simulink model "ACC_COM"  (R2022b)
settings: configuration reference "ACC_AutosarConfig" (kept outside this file)
model workspace (MATLAB code in the model file):
  | cmdLim = Simulink.Parameter;
  | cmdLim.Value = 15;
  | cmdLim.Description = 'Limit for controlling the maximum surface command angle.';
  | cmdLim.Min = 0;
  | cmdLim.Max = 90;
  | cmdLim.DocUnits = 'deg';
  | 
  | dispGain = Simulink.Parameter;
  | dispGain.Value = 0.75;
  | dispGain.Description = 'Gain applied to the displacement error.';
  | dispGain.Min = 0;
  | dispGain.Max = [];
  | dispGain.DocUnits = 'deg/sec/deg';
  | 
  | dispLim = Simulink.Parameter;
  | dispLim.Value = 30;
  | dispLim.Description = 'Limit for controlling the maximum commanded angle.';
  | dispLim.Min = 0;
  | dispLim.Max = 180;
  | dispLim.DocUnits = 'deg';
  | 
  | intGain = Simulink.Parameter;
  | intGain.Value = 0.5;
  | intGain.Description = 'Gain applied to the integral error.';
  | intGain.Min = 0;
  | intGain.Max = [];
  | intGain.DocUnits = 'deg/sec/deg/sec';
  | 
  | intLim = Simulink.Parameter;
  | intLim.Value = 5;
  | intLim.Description = 'Limit for controlling the maximum commanded angle.';
  | intLim.Min = 0;
  | intLim.Max = 90;
  | intLim.DocUnits = 'deg';
  | 
  | rateGain = Simulink.Parameter;
  | rateGain.Value = 2;
  | rateGain.Description = 'Gain applied to the rate error.';
  | rateGain.Min = 0;
  | rateGain.Max = [];
  | rateGain.DocUnits = 'deg/deg/sec';
  | 
  | rateLim = Simulink.Parameter;
  | rateLim.Value = 6;
  | rateLim.Description = 'Limit for controlling the maximum commanded angle.';
  | rateLim.Min = 0;
  | rateLim.Max = 180;
  | rateLim.DocUnits = 'deg/sec';
  | 
  | hdgGain = Simulink.Parameter;
  | hdgGain.Value = 0.015;
values from neighbouring files (symbols this model uses):
  ACC_SampleTime = 0.01    [ACC_DD.sldd]
settings Model: RequirementInfo={} %GIDa_fe9045fd_0412_4b6e_8206_617cc20e6fde  DataDictionary=ACC_DD.sldd  FPTRunName=Active  Creator=MAAM  LastModifiedBy=MAAM
settings ConfigSetRef: SourceName=ACC_AutosarConfig

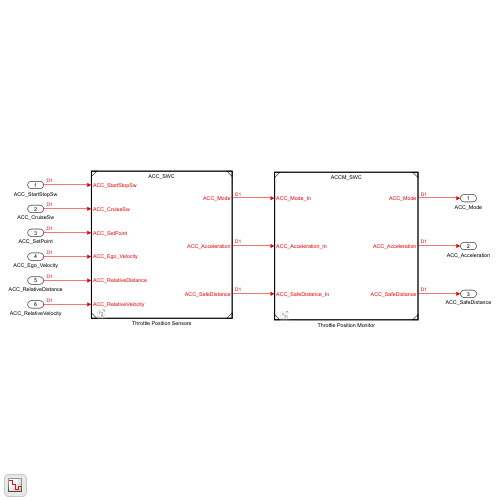
[thumbnail: Simulink's stored preview of the top-level diagram]
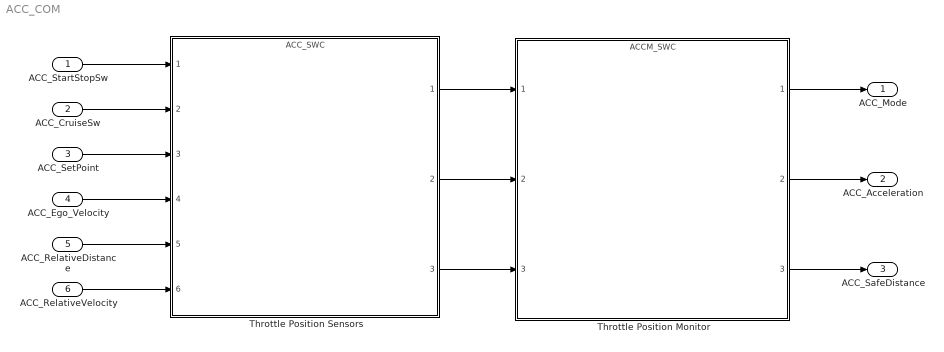
== system ACC_COM ==
  ACC_StartStopSw : Inport  OutDataTypeStr=boolean  SampleTime=ACC_SampleTime
  ACC_CruiseSw : Inport  Port=2  OutDataTypeStr=boolean  SampleTime=ACC_SampleTime
  ACC_SetPoint : Inport  Port=3  OutDataTypeStr=single  SampleTime=ACC_SampleTime
  ACC_Ego_Velocity : Inport  Port=4  OutDataTypeStr=single  SampleTime=ACC_SampleTime
  ACC_RelativeDistance : Inport  Port=5  OutDataTypeStr=single  SampleTime=ACC_SampleTime
  ACC_RelativeVelocity : Inport  Port=6  OutDataTypeStr=single  SampleTime=ACC_SampleTime
  Throttle Position Monitor : ModelReference  ModelNameDialog=ACCM_SWC.slx  SimulationMode=Normal  ModelReferenceVersion=1.7
  Throttle Position Sensors : ModelReference  ModelNameDialog=ACC_SWC.slx  SimulationMode=Normal  ModelReferenceVersion=1.6
  ACC_Mode : Outport
  ACC_Acceleration : Outport  Port=2
  ACC_SafeDistance : Outport  Port=3
  wires:
  ACC_StartStopSw/1 -> Throttle Position Sensors/1
  ACC_CruiseSw/1 -> Throttle Position Sensors/2
  ACC_SetPoint/1 -> Throttle Position Sensors/3
  ACC_Ego_Velocity/1 -> Throttle Position Sensors/4
  ACC_RelativeDistance/1 -> Throttle Position Sensors/5
  ACC_RelativeVelocity/1 -> Throttle Position Sensors/6
  Throttle Position Monitor/2 -> ACC_Acceleration/1
  Throttle Position Monitor/3 -> ACC_SafeDistance/1
  Throttle Position Sensors/1 -> Throttle Position Monitor/1
  Throttle Position Sensors/2 -> Throttle Position Monitor/2
  Throttle Position Sensors/3 -> Throttle Position Monitor/3
  Throttle Position Monitor/1 -> ACC_Mode/1
